simulink library "CTRL_LO_ST1_WHFSUM"  (R2023b)
settings: Solver=VariableStepAuto  StartTime=0.0  StopTime=10.0  RelTol=1e-3
settings Model: Creator=blatak  LastModifiedBy=blatak

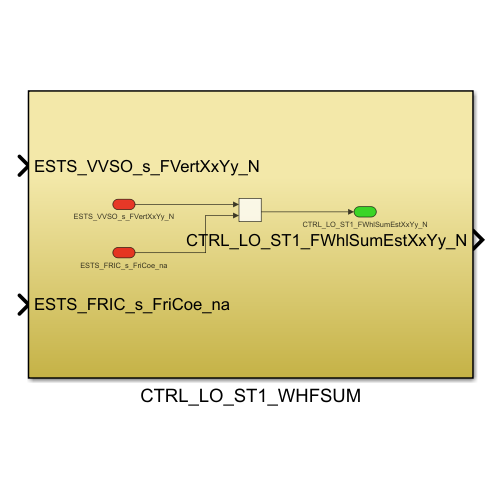
[thumbnail: Simulink's stored preview of the top-level diagram]
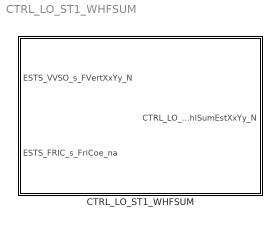
== system CTRL_LO_ST1_WHFSUM ==
  CTRL_LO_ST1_WHFSUM : Subsystem

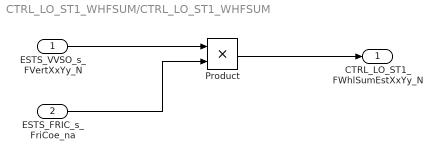
== system CTRL_LO_ST1_WHFSUM/CTRL_LO_ST1_WHFSUM ==
  ESTS_VVSO_s_FVertXxYy_N : Inport
  ESTS_FRIC_s_FriCoe_na : Inport  Port=2
  Product : Product
  CTRL_LO_ST1_FWhlSumEstXxYy_N : Outport
  wires:
  ESTS_VVSO_s_FVertXxYy_N/1 -> Product/1
  ESTS_FRIC_s_FriCoe_na/1 -> Product/2
  Product/1 -> CTRL_LO_ST1_FWhlSumEstXxYy_N/1
